simulink library "AEMS_Standard_Library"  (R2016b)
settings: Solver=ode45  StartTime=0.0  StopTime=10.0  RelTol=1e-3
undefined symbols (not defined in the file or in its folder): BkPY, carto, Cbx_extegr, Cbx_lpegrsys, Cbx_portegr, Cnx_bnk_nr_conf, Cnx_cyl_nr_conf, ConfigManagement, configuration_management, Cxx_dcm_io_tmr_end_xxxx, Cxx_dcm_rt_tmr_end, Cxx_DID_xxxx_IO_max, Cxx_DID_xxxx_IO_min, Cxx_egrhsofs, Cxx_vmaniegi, DEM_DEBOUNCE_FREEZE, DEM_DTR_CTL_INVISIBLE, DEM_DTR_CTL_NORMAL, Dem_DtrId2_XXX, Dem_DtrId3_XXX, Dem_DtrId4_XXX, Dem_DtrId5_XXX, Dem_DtrId6_XXX, Dem_DtrId7_XXX, Dem_DtrId8_XXX, Dem_DtrId9_XXX, Dem_DtrId_XXX, Dem_EnableConditionId2_XXX, Dem_EnableConditionId3_XXX, Dem_EnableConditionId4_XXX, Dem_EnableConditionId5_XXX, Dem_EnableConditionId6_XXX, Dem_EnableConditionId7_XXX, Dem_EnableConditionId8_XXX, Dem_EnableConditionId_XXX, Dem_EventId, Dem_EventId2_XXX, Dem_EventId3_XXX, Dem_EventId4_XXX, Dem_EventId5_XXX, Dem_EventId6_XXX, Dem_EventId7_XXX, Dem_EventId8_XXX, Dem_EventId9_XXX, Dem_EventId_Device_Faulttype, Dem_EventId_XXX, DEM_IUMPR_GENERAL_DENOMINATOR, DEM_OPCYC_IGNITION, Dem_RatioId2_XXX, Dem_RatioId3_XXX, Dem_RatioId4_XXX, Dem_RatioId5_XXX, Dem_RatioId6_XXX, Dem_RatioId7_XXX, Dem_RatioId8_XXX, Dem_RatioId_XXX, Dem_StorageConditionId2_XXX, Dem_StorageConditionId3_XXX, Dem_StorageConditionId4_XXX, Dem_StorageConditionId5_XXX ... (+65)
libraries: AEMS_Standard_Library x477, simulink x2
(part 8 of 39)

== system AEMS_Standard_Library/DISCONTINUITIES ==
  AEMS_DEADZONE : Subsystem  Tag=[LIB]  mask(AEMS_DEADZONE){mf=off}
      mask prompts: mf "Curve inflexion dead-zone"
      mask help:
      | Outputs zero for inputs within the dead zone.
      | Offset input signals by either the Start(lowerlimit) or End(upperlimit) value when the input is outside the dead zone.
      |
      | 'Start' is the lower dead-zone boundary.
      | 'End' is the upper dead-zone boundary.
      |
      | For 'Curve inflexion dead-zone' checked OFF, the output signal has three phases based on input signal VALUE:
      |
      | 1] When input signal is below the 'start' boundary, the output signal has an offset of - 'start'.
      | 2] When input signal is above the 'end' boundary, the output signal has an offset of - 'end'.
      | 3] When input signal is between the 'start' and 'end' boundaries, the output signal is set to ZERO
      |
      | For 'Curve inflexion dead-zone' checked ON, the output signal has three phases based on input signal VALUE and its DERIVATIVE (with respect to time):
      |
      | 1] When input signal derivative is positive (and remains positive), the output signal has an offset of - 'start'.
      | 2] When input signal derivative is negative (and remains negative), the output signal has an offset of - 'end'.
      | 3] When input signal derivative changes sign, the output signal keeps its last value until it has an offset of  - 'start' (for a - to + change) or - 'end' (for a + to - change).
      mask init:
      | if mf
      |     patch_out=[0,.1,.4,.6,.8,1,1,.8,.6,.4,.1,0;.19,.19,.49,.49,.29,.29,.31,.31,.51,.51,.21,.21];
      | else
      |     patch_out=[0,.1,.3,.4,.5,.7,.8,.9,1,1,.9,.8,.7,.5,.4,.3,.1,0;.29,.39,.39,.49,.39,.39,.29,.39,.39,.41,.41,.31,.41,.41,.51,.41,.41,.31];
      | end
      settings: AttributesFormatString=%<MaskType>\nCurve inflexion dead-zone = %<mf>
      mask Help:
      | eval('path_lib=fileparts(which(''AEMS_Standard_Library''));');
      | doc_path = [path_lib '\help\AEMS_DEADZONE.pdf'];
      | eval('open(doc_path)');
      mask Display:
      | patch([0,.4,.8,1,1,.8,.4,0],[.19,.59,.19,.39,.41,.21,.61,.21],[0 0 1])
      | 
      | patch(patch_out(1,:),patch_out(2,:),[1 0 0])
      | 
      | 
      | plot([0.02,0.02,0.02])
      | plot([0.98,0.98,0.98])
      | 
      | text(0.5, 0.15, 'AEMS_DEADZONE', 'horizontalAlignment', 'center');
  AEMS_ENUMERATION_SWITCH : Subsystem  Tag=[LIB]  mask(AEMS_ENUMERATION_SWITCH){DataPortIndices={[Nnx_aaa_stt, Nnx_bbb_stt] ,Nnx_ccc_stt,Nnx_ddd_stt}, DataPortForDefault=Last data port}
      mask prompts: DataPortIndices "Data Port Indices"; DataPortForDefault "Data port for default case"
      mask help: Custom multiport switch block to display enum constant names on the mask.
      mask init:
      | % To mask the Multiport Switch block
      | 
      | %% Getting parameter data
      | ThisBlk=gcb;
      | DPI_tmp=get_param(ThisBlk,'DataPortIndices');
      | DPI = regexprep(DPI_tmp,'\s','');
      | DPDC=get_param(ThisBlk,'DataPortForDefault');
      | 
      | %% CHECK PART
      | % If parameters are the same, do nothing
      | Internal_DPI=get_param([ThisBlk '/MultiportSwitch'],'DataPortIndices');
      | Internal_DPDC=get_param([ThisBlk '/MultiportSwitch'],'DataPortForDefault');
      | if strcmp(DPI,Internal_DPI) && strcmp(DPDC,Internal_DPDC) 
      |     return
      | end
      | 
      | % Test if some parameters are in duplicate
      | DPI_complete=strsplit(regexprep(DPI,'{|}|\[|\]',''),',');
      | DPI_unique = unique(DPI_complete,'stable');
      | if ~isequal(DPI_complete,DPI_unique)
      |     msgbox('Invalid setting for data port indices. The same Nnx is used more than once','Error','error');
      |     return
      | end
      | 
      | % Test if some parameters are not Nnx_stt
      | if ~all(startsWith(DPI_complete,'Nnx')) || ~all(endsWith(DPI_complete,'_stt'))
      |     msgbox('Data port indices should start with ''Nnx'' and end with ''stt''','Error','error');
      |     return
      | end
      | 
      | %% MODIFICATION OF INNER PART
      | 
      | 
      | % Total number of inports we need inside incl. default case
      | TargetInports = regexp(DPI,'(\w+)|\[([^\[\]]*)\]','tokens');
      | if isequal(DPDC,'Additional data port')
      |     TargetInports_Nb = numel(TargetInports)+1;
      | else
      |     TargetInports_Nb = numel(TargetInports);
      | end
      | 
      | % Total number of existing inports
      | ExistingInports=find_system(ThisBlk,'LookUnderMasks','all','FollowLinks','on','regexp','on','BlockType','Inport','Name','^Dataport');
      | ExistingInports_Nb = length(ExistingInports);
      | 
      | % If we need to create inports and their lines
      | if TargetInports_Nb > ExistingInports_Nb    
      |         % creating blocks
      |         PreviousInportPosition=get_param([ThisBlk '/Dataport' num2str(ExistingInports_Nb)],'Position');
      |         for num=ExistingInports_Nb:(TargetInports_Nb-1)
      |             NewInportPosition=[10   PreviousInportPosition(2)+35    40   PreviousInportPosition(4)+35];
      |             add_block('built-in/Inport',[ThisBlk '/Dataport' num2str(num+1)],'Position',NewInportPosition,'BackgroundColor','green');
      |             PreviousInportPosition(2)= NewInportPosition(2);
      |             PreviousInportPosition(4)= NewInportPosition(4);
      |         end
      | % If we need to delete inports and their lines
      | elseif TargetInports_Nb < ExistingInports_Nb
      |         for num=(TargetInports_Nb):ExistingInports_Nb-1
      |             delete_block([ThisBlk '/Dataport' num2str(num+1)]);
      |         end
      | end
      | 
      | % We set the parameters of the inner block to the new ones
      | % Script may fail here if a data is not defined
      | try
      |     set_param([ThisBlk,'/MultiportSwitch'],'DataPortForDefault',DPDC,'DataPortIndices',DPI);
      | 
      |     % deleting all lines then creating all lines
      |     delete_line(find_system(ThisBlk,'FindAll','on','FollowLinks','on','LookUnderMasks','all','Type','line'));
      |     add_line(ThisBlk,'Control_Input/1','MultiportSwitch/1','Autorouting','On');
      |     add_line(ThisBlk,'MultiportSwitch/1','Out/1','Autorouting','On');
      |     for num=0:(TargetInports_Nb-1)
      |         add_line(ThisBlk,['Dataport' num2str(num+1) '/1'],['MultiportSwitch/' num2str(num+2)],'Autorouting','On');
      |     end
      | catch
      | end
      settings: AttributesFormatString=%<MaskType>\nData port for default case = %<DataPortForDefault>
      mask Help:
      | eval('path_lib=fileparts(which(''AEMS_Standard_Library''));');
      | doc_path = [path_lib '\help\AEMS_ENUMERATION_SWITCH.pdf'];
      | eval('open(doc_path)');
      mask TypeOptions DataPortForDefault: Last data port | Additional data port
      mask Display:
      | % To mask the Multiport Switch block
      | 
      | %% Getting parameter data
      | ThisBlk=gcb;
      | DPI = get_param(ThisBlk,'DataPortIndices');
      | DPI = regexprep(DPI,'\s','');
      | DPDC=get_param(ThisBlk,'DataPortForDefault');
      | 
      | 
      | %% CHECK PART
      | % Test if some parameters are in duplicate
      | DPI_complete=strsplit(regexprep(DPI,'{|}|\[|\]',''),',');
      | DPI_unique = unique(DPI_complete,'stable');
      | if ~isequal(DPI_complete,DPI_unique)
      |    disp('!!! Invalid Settings !!!\nDuplicate Nnx');
      |    return
      | end
      | 
      | % Test if some parameters are not Nnx_stt
      | if ~all(startsWith(DPI_complete,'Nnx')) || ~all(endsWith(DPI_complete,'_stt'))
      |    disp('!!! Invalid Settings !!!\nNot all Nnx_..._stt constants');
      |    return
      | end
      | 
      | 
      | %%DRAWING PART
      | Blkpos = get_param(ThisBlk,'Position');
      | PortHandles=get_param(gcb,'PortHandles');
      | IPort_Pos=get_param(PortHandles.Inport,'Position');
      | BlockHeightPx = Blkpos(4)-Blkpos(2);
      | 
      | %% drawing inputs
      | % splitting fileds in inputs
      | Inputs_ToDraw = regexp(DPI,'(\w+)|\[([^\[\]]*)\]','tokens');
      | 
      | % adding carriage returns every two Nnx in case there in several per input,
      | % and spaces after each comma
      | Inputs_ToDraw=cellfun(@(x) regexprep(x,'(\w+\,\w+\,)','$1\n'),Inputs_ToDraw,'UniformOutput',0);
      | Inputs_ToDraw=cellfun(@(x) regexprep(x,'(\w+)\,','$1, '),Inputs_ToDraw,'UniformOutput',0);
      | 
      | Input_YPos=cellfun(@(x) (Blkpos(4)-x(2))/BlockHeightPx,IPort_Pos,'UniformOutput',0);
      | for i=2:(numel(Input_YPos))
      |     x=[-0.1,0.4];
      |     y=[Input_YPos{i},Input_YPos{i}];
      |     plot(x,y);
      | 
      |     if i==numel(Input_YPos)
      |         if isequal(DPDC,'Additional data port')
      |             port_label('input', i, ['*' sprintf('\n')]);
      |         else
      |             port_label('input', i, ['*, ' char(Inputs_ToDraw{i-1}) sprintf('\n')]);
      |         end
      |     else
      |         port_label('input', i, [char(Inputs_ToDraw{i-1}) sprintf('\n')]);
      |     end
      | end
      | 
      | %% draw selector lines
      | x=[-0.1 0.3];
      | y=[Input_YPos{1},Input_YPos{1}];
      | plot(x,y);
      | x=[0.3,0.3];
      | y=[Input_YPos{1}+0.04,Input_YPos{1}-0.04];
      | plot(x,y);
      | 
      | %% draw output lines
      | XPlot_Line = [0.43,0.8,1.1];
      | YPlot_Line = [Input_YPos{2},0.5,0.5];
      | plot(XPlot_Line,YPlot_Line);
  AEMS_MULTI_PORT_TIME_SWITCH : Subsystem  Tag=[LIB]  mask(AEMS_MULTI_PORT_TIME_SWITCH){}
      mask help:
      | This switch allows the user to switch among 8 input signals using the Vsx_sel input. It provides a smooth transition between the previously selected signal and the currently selected signal over a period of time, set by Vxx_swi_t.
      |
      | It should be noted that during the transition, the current value of both signals is taken into account and not just values at the moment of switching.
      |
      | As a result, discontinuities can arise if a new signal is seleted before the previous transition has ended.
      settings: AttributesFormatString=%<MaskType>
      mask Help:
      | eval('path_lib=fileparts(which(''AEMS_Standard_Library''));');
      | doc_path = [path_lib '\help\AEMS_MULTI_PORT_TIME_SWITCH.pdf'];
      | eval('open(doc_path)')
      mask Display: disp('AEMS_MULTI_PORT_TIME_SWITCH')
  AEMS_SLEW_RATE : Subsystem  Tag=[LIB]  mask(AEMS_SLEW_RATE){}
      mask help:
      | This block is a Slew rate block, which limits the increase and decrease of the INPUT by using calibrated slopes independent of sampling time.
      | POS_SLOPE : positive maximum slope parameter per second.
      | NEG_SLOPE : negative maximum slope parameter per second.
      |
      | Reference to AUTOSAR specification:
      | AUTOSAR Service Name : Mfl_RampCalc
      | Reference : SWS_Mfl_00201
      settings: AttributesFormatString=%<MaskType>
      mask Help:
      | eval('path_lib=fileparts(which(''AEMS_Standard_Library''));');
      | doc_path = [path_lib '\help\AEMS_SLEW_RATE.pdf'];
      | eval('open(doc_path)')
      mask Display:
      | patch([0.1 0.2 0.22 0.25 0.3 0.35 0.4 0.45 0.5 0.6 0.6 0.5 0.45 0.4 0.35 0.3 0.25 0.22 0.2 0.1],[0.24 0.24 0.34 0.44 0.59 0.69 0.79 0.84 0.89 0.89 0.93 0.93 0.88 0.83 0.73 0.63 0.48 0.38 0.28 0.28],[0 0 1]);
      | patch([0.5 0.6 0.65 0.68 0.72 0.79 0.8 0.9 0.9 0.8 0.79 0.72 0.68 0.65 0.6 0.5],[0.89 0.89 0.76 0.71 0.67 0.65 0.64 0.64 0.68 0.68 0.69 0.71 0.75 0.8 0.93 0.93],[0 0 1])
      | patch([0.1 0.2 0.5 0.6 0.8 0.9 0.9 0.8 0.6 0.5 0.2 0.1],[0.25 0.25 0.9 0.9 0.65 0.65 0.67 0.67 0.92 0.92 0.27 0.27],[1 0 0]);
  AEMS_SLOPE_SWITCH : Subsystem  Tag=[LIB]  mask(AEMS_SLOPE_SWITCH){}
      mask help:
      | This block is a Multiple Port Slope Switch.
      | Depending on the value of input Switch_Cmd (from 0), the block outputs the corresponding input signal.
      | For Switch_Cmd = 0, Output is In0, for Switch_Cmd = 1, Output is In1, and so on...
      |
      | Nevertheless, for each switch between two input signals, a slope is activated from the first input signal to the second input signal.
      | The value of this slope is given by Pos_Slope if the input signal to reach is over the initial input signal and by Neg_Slope if the input signal to reach is under.
      | Pos_Slope and Neg_Slope are respectively the positive and negative slope parameters per second.
      |
      | The output Slope_On indicates if a transition is active (Slope_On at true) or not (Slope_On at false).
      settings: AttributesFormatString=%<MaskType>
      mask Help:
      | eval('path_lib=fileparts(which(''AEMS_Standard_Library''));');
      | doc_path = [path_lib '\help\AEMS_SLOPE_SWITCH.pdf'];
      | eval('open(doc_path)')
      mask Display:
      | color ('blue')
      | disp('SLOPE SWITCH\n\n 2 INPUTS')
  AEMS_SLOPE_SWITCH_3INPUTS : Subsystem  Tag=[LIB]  mask(AEMS_SLOPE_SWITCH_3INPUTS){}
      mask help:
      | This block is a Multiple Port Slope Switch.
      | Depending on the value of input Switch_Cmd (from 0), the block outputs the corresponding input signal.
      | For Switch_Cmd = 0, Output is In0, for Switch_Cmd = 1, Output is In1, and so on...
      |
      | Nevertheless, for each switch between two input signals, a slope is activated from the first input signal to the second input signal.
      | The value of this slope is given by Pos_Slope if the input signal to reach is over the initial input signal and by Neg_Slope if the input signal to reach is under.
      | Pos_Slope and Neg_Slope are respectively the positive and negative slope parameters per second.
      |
      | The output Slope_On indicates if a transition is active (Slope_On at true) or not (Slope_On at false).
      settings: AttributesFormatString=%<MaskType>
      mask Help:
      | eval('path_lib=fileparts(which(''AEMS_Standard_Library''));');
      | mskblk=get_param(gcbh,'MaskType');
      | doc_path = [path_lib '\help\',mskblk,'.pdf'];
      | eval('open(doc_path)');
      mask Display:
      | color ('blue')
      | disp('SLOPE SWITCH\n\n 3 INPUTS')
  AEMS_SLOPE_SWITCH_4INPUTS : Subsystem  Tag=[LIB]  mask(AEMS_SLOPE_SWITCH_4INPUTS){}
      mask help:
      | This block is a Multiple Port Slope Switch.
      | Depending on the value of input Switch_Cmd (from 0), the block outputs the corresponding input signal.
      | For Switch_Cmd = 0, Output is In0, for Switch_Cmd = 1, Output is In1, and so on...
      |
      | Nevertheless, for each switch between two input signals, a slope is activated from the first input signal to the second input signal.
      | The value of this slope is given by Pos_Slope if the input signal to reach is over the initial input signal and by Neg_Slope if the input signal to reach is under.
      | Pos_Slope and Neg_Slope are respectively the positive and negative slope parameters per second.
      |
      | The output Slope_On indicates if a transition is active (Slope_On at true) or not (Slope_On at false).
      settings: AttributesFormatString=%<MaskType>
      mask Help:
      | eval('path_lib=fileparts(which(''AEMS_Standard_Library''));');
      | doc_path = [path_lib '\help\AEMS_SLOPE_SWITCH_4INPUTS.pdf'];
      | eval('open(doc_path)')
      mask Display:
      | color ('blue')
      | disp('SLOPE SWITCH\n\n 4 INPUTS')
  AEMS_SLOPE_SWITCH_6INPUTS : Subsystem  Tag=[LIB]  mask(AEMS_SLOPE_SWITCH_6INPUTS){}
      mask help:
      | This block is a Multiple Port Slope Switch.
      | Depending on the value of input Switch_Cmd (from 0), the block outputs the corresponding input signal.
      | For Switch_Cmd = 0, Output is In0, for Switch_Cmd = 1, Output is In1, and so on...
      |
      | Nevertheless, for each switch between two input signals, a slope is activated from the first input signal to the second input signal.
      | The value of this slope is given by Pos_Slope if the input signal to reach is over the initial input signal and by Neg_Slope if the input signal to reach is under.
      | Pos_Slope and Neg_Slope are respectively the positive and negative slope parameters per second.
      |
      |
      | The output Slope_On indicates if a transition is active (Slope_On at true) or not (Slope_On at false).
      settings: AttributesFormatString=%<MaskType>
      mask Help:
      | eval('path_lib=fileparts(which(''AEMS_Standard_Library''));');
      | mskblk=get_param(gcbh,'MaskType');
      | doc_path = [path_lib '\help\',mskblk,'.pdf'];
      | eval('open(doc_path)');
      mask Display:
      | color ('blue')
      | disp('SLOPE SWITCH\n\n 6 INPUTS')
  AEMS_SLOPE_SWITCH_8INPUTS : Subsystem  Tag=[LIB]  mask(AEMS_SLOPE_SWITCH_8INPUTS){}
      mask help:
      | This block is a Multiple Port Slope Switch.
      | Depending on the value of input Switch_Cmd (from 0), the block outputs the corresponding input signal.
      | For Switch_Cmd = 0, Output is In0, for Switch_Cmd = 1, Output is In1, and so on...
      |
      | Nevertheless, for each switch between two input signals, a slope is activated from the first input signal to the second input signal.
      | The value of this slope is given by Pos_Slope if the input signal to reach is over the initial input signal and by Neg_Slope if the input signal to reach is under.
      | Pos_Slope and Neg_Slope are respectively the positive and negative slope parameters per second.
      |
      |
      | The output Slope_On indicates if a transition is active (Slope_On at true) or not (Slope_On at false).
      settings: AttributesFormatString=%<MaskType>
      mask Help:
      | eval('path_lib=fileparts(which(''AEMS_Standard_Library''));');
      | doc_path = [path_lib '\help\AEMS_SLOPE_SWITCH_8INPUTS.pdf'];
      | eval('open(doc_path)')
      mask Display:
      | color ('blue')
      | disp('SLOPE SWITCH\n\n 8 INPUTS')

== system AEMS_Standard_Library/DISCRETE ==
  AEMS_UNITDELAY_EXTERNALIC : Subsystem  Tag=[LIB]  mask(AEMS_UNITDELAY_EXTERNALIC){}
      mask help:
      | The input signal (u) signal will be delayed by one sample period and given as output (y).
      | Initial condition is given by the signal IC.
      |
      | Note: Input must be without offset
      settings: AttributesFormatString=%<MaskType>
      mask Help:
      | eval('path_lib=fileparts(which(''AEMS_Standard_Library''));');
      | doc_path = [path_lib '\help\AEMS_UNITDELAY_EXTERNALIC.pdf'];
      | eval('open(doc_path)')
      mask Display: dpoly(1,[1 0],'z')
  AEMS_UNITDELAY_RESET_EXTERNALIC : Subsystem  Tag=[LIB]  mask(AEMS_UNITDELAY_RESET_EXTERNALIC){}
      mask help:
      | The output is the signal (u) delayed by one sample period.
      | When the reset signal 'R' is true, the state and the output are always set equal to the initial condition signal 'IC'.  This reset action is vectorized and supports scalar expansion.
      settings: AttributesFormatString=%<MaskType>
      mask Help:
      | eval('path_lib=fileparts(which(''AEMS_Standard_Library''));');
      | doc_path = [path_lib '\help\AEMS_UNITDELAY_RESET_EXTERNALIC.pdf'];
      | eval('open(doc_path)')
      mask Display: dpoly(1,[1 0],'z')

== system AEMS_Standard_Library/EDGE ==
  AEMS_EDGE_EITHER : Subsystem  Tag=[LIB]  mask(AEMS_EDGE_EITHER){init=false}
      mask prompts: init "Initial Value of Input"
      mask help:
      | This block can be used to :
      |
      | Detect change   - If the input signal(In) is changing from '0' to '1' OR '1' to '0'
      |
      | The initial value of Input is given in the mask. By default it gets value FALSE.
      |
      | The output is a signal of data type 'boolean'.
      |
      | Reference to AUTOSAR specification:
      |         AUTOSAR Service Name :  Efx_EdgeBipol_u8_u8
      |         Reference : SWS_Efx_00380
      mask init:
      | a=0.2;
      | b=0.4;
      | c=0.6;
      | d=0.9;
      | e=0.6;
      | f=0.6;
      | g=0.9;
      | if strcmp(init,'false')
      |    InitValue=0;
      | elseif strcmp(init,'true')
      |    InitValue=1; 
      | end
      settings: AttributesFormatString=|
      | %<MaskType>
      | Initial Value : %<init>
      mask Help:
      | eval('path_lib=fileparts(which(''AEMS_Standard_Library''));');
      | mskblk=get_param(gcbh,'MaskType');
      | doc_path = [path_lib '\help\',mskblk,'.pdf'];
      | eval('open(doc_path)');
      mask TypeOptions init: false | true
      mask DialogControl DescGroupVar_copy Prompt: Initialization
      mask Display:
      | color('green');
      | plot([a b b c],[f f g g]);
      | color('red');
      | plot([a b b c],[d d e e]);
      | color('blue');
      | plot([a b b b c],[0.1 0.1 0.4 0.1 0.1])
  AEMS_EDGE_FALLING : Subsystem  Tag=[LIB]  mask(AEMS_EDGE_FALLING){init=false}
      mask prompts: init "Initial Value of Input"
      mask help:
      | This block can be used to :
      |
      | Detect decrease - If the input signal(In) is changing from '1' to '0'.
      |
      | The initial value of Input is given in the mask. By default it gets value FALSE.
      |
      | The output is a signal of data type 'boolean'.
      |
      | Reference to AUTOSAR specification:
      |          AUTOSAR Service Name :  Efx_EdgeFalling_u8_u8
      |          Reference : SWS_Efx_00382
      mask init:
      | a=0.2;
      | b=0.4;
      | c=0.6;
      | d=0.9;
      | e=0.6;
      | f=0.9;
      | g=0.6;
      | if strcmp(init,'false')
      |    InitValue=0;
      | elseif strcmp(init,'true')
      |    InitValue=1; 
      | end
      settings: AttributesFormatString=|
      | %<MaskType>
      | Initial Value : %<init>
      mask Help:
      | eval('path_lib=fileparts(which(''AEMS_Standard_Library''));');
      | mskblk=get_param(gcbh,'MaskType');
      | doc_path = [path_lib '\help\',mskblk,'.pdf'];
      | eval('open(doc_path)');
      mask TypeOptions init: false | true
      mask Display:
      | color('green');
      | plot([a b b c],[f f g g]);
      | color('red');
      | plot([a b b c],[d d e e]);
      | color('blue');
      | plot([a b b b c],[0.1 0.1 0.4 0.1 0.1])
  AEMS_EDGE_RISING : Subsystem  Tag=[LIB]  mask(AEMS_EDGE_RISING){init=false}
      mask prompts: init "Initial Value of Input"
      mask help:
      | This block can be used to :
      |
      | Detect increase - If the input signal(In) is changing from '0' to '1'.
      |
      | The initial value of Input is given in the mask. By default it gets value FALSE.
      |
      | The output is a signal of data type 'boolean'.
      |
      | Reference to AUTOSAR specification:
      |         AUTOSAR Service Name :  Efx_EdgeRising_u8_u8
      |         Reference : SWS_Efx_00384
      mask init:
      | %Rising
      | a=0.2;
      | b=0.4;
      | c=0.6;
      | d=0.6;
      | e=0.9;
      | f=0.6;
      | g=0.9;
      | if strcmp(init,'false')
      |    InitValue=0;
      | elseif strcmp(init,'true')
      |    InitValue=1; 
      | end
      settings: AttributesFormatString=|
      | %<MaskType>
      | Initial Value : %<init>
      mask Help:
      | eval('path_lib=fileparts(which(''AEMS_Standard_Library''));');
      | mskblk=get_param(gcbh,'MaskType');
      | doc_path = [path_lib '\help\',mskblk,'.pdf'];
      | eval('open(doc_path)');
      mask TypeOptions init: false | true
      mask Display:
      | color('green');
      | plot([a b b c],[f f g g]);
      | color('red');
      | plot([a b b c],[d d e e]);
      | color('blue');
      | plot([a b b b c],[0.1 0.1 0.4 0.1 0.1])

== system AEMS_Standard_Library/FILTER ==
  AEMS_DISCRETE_TIME_INTEGRATOR_EULER : Subsystem  Tag=[LIB]  mask(AEMS_DISCRETE_TIME_INTEGRATOR_EULER){Upper_limit=255, Lower_limit=0}
      mask prompts: Upper_limit "Upper Saturation Limt"; Lower_limit "Lower Saturation Limit"
      mask help:
      | The block can integrate or accumulate using the Forward Euler.
      | The resulting expression for the output of the block at step n is
      | y(n) = x(n-1)*T*K + y(n-1)
      settings: AttributesFormatString=%<MaskType>\nUpper Saturation Limit = %<Upper_limit>\nLower Saturation Limit = %<Lower_limit>
      mask Help:
      | eval('path_lib=fileparts(which(''AEMS_Standard_Library''));');
      | doc_path = [path_lib '\help\AEMS_DISCRETE_TIME_INTEGRATOR_EULER.pdf'];
      | eval('open(doc_path)')
      mask Display: disp('Discrete-Time \n Integrator')
  AEMS_FILTER_WITH_DELAY_CONTROL : Subsystem  Tag=[LIB]  mask(AEMS_FILTER_WITH_DELAY_CONTROL){}
      mask help:
      | The principle of this filter is based on slopes limitation of the signal to process.
      | The set points to limit the negative and positive slopes are computed with the derivate of the input filtered signal using a low pass first order filter.
      | The set points are then fixed by a proportional integrator controller in order to minimize the error between the input and output.
      |
      | Notes: filter_param is calculated from time constant and sample time as:
      | filter_param=1-exp(-T/Tau) where T is sample time and Tau is time constant.
      |
      | See Help document for more information.
      settings: AttributesFormatString=%<MaskType>
      mask Help:
      | eval('path_lib=fileparts(which(''AEMS_Standard_Library''));');
      | doc_path = [path_lib '\help\AEMS_FILTER_WITH_DELAY_CONTROL.pdf'];
      | eval('open(doc_path)')
      mask Display:
      | port_label('input',1,'filter_param')
      | port_label('input',2,'kp')
      | port_label('input',3,'Input')
      | port_label('input',4,'timestep')
      | port_label('output',1,'Output')
      | disp('AEMS_FILTER_WITH_DELAY_CONTROL')
  AEMS_FIRST_ORDER_FILTER_RST : Subsystem  Tag=[LIB]  mask(AEMS_FIRST_ORDER_FILTER_RST){}
      mask help:
      | This block is a First-Order Filter, with :
      | 	- Filter_param: filter parameter calculated from time constant and sample time.
      | 	- IC the initial value.
      | 	- R the reset signal.
      | The initial condition is given by the signal IC.
      | When the reset signal is true, output is set equal to the initial condition signal IC.
      |
      | Notes: Filter_param is calculated from time constant and sample time as:
      | Filter_param=1-exp(-T/Tau) where T is sample time and Tau is time constant.
      |
      | Reference to AUTOSAR specification:
      | -	AUTOSAR Service Name:  Efx_LpFilter
      | -	Reference: [SWS_Efx_00012]
      |
      | See Help document for more information.
      settings: AttributesFormatString=%<MaskType>
      mask Help:
      | eval('path_lib=fileparts(which(''AEMS_Standard_Library''));');
      | mskblk=get_param(gcbh,'MaskType');
      | doc_path = [path_lib '\help\',mskblk,'.pdf'];
      | eval('open(doc_path)');
      mask Display:
      | plot([0.2  0.2],[0.1 0.9 ]);
      | plot([0.25  0.2],[0.8 0.9 ]);
      | plot([0.15  0.2],[0.8 0.9 ]);
      | plot([0.9  0.2],[0.8 0.8 ]);
      | plot([0.2  1],[0.1 0.1 ]);
      | plot([0.2:0.01:0.85],0.1+0.7-0.7*exp(5*[0:-0.01:-.65]));
      | plot([1  0.9],[0.1 0.15]);
      | plot([1  0.9],[0.1 0.05]);
  AEMS_FORWARD_EULER_INTEGRATOR_WITH_RESET : Subsystem  Tag=[LIB]  mask(AEMS_FORWARD_EULER_INTEGRATOR_WITH_RESET){}
      mask help:
      | This block will perform discrete-time integration or accumulation of input signal based on Euler's method :
      | y[k] = y[k-1] + K.Ts.u[k-1]
      |
      |  Where,
      |  K = gain
      |  Ts = sample time.
      |  IC = initial condition.
      |
      | Output(y) will be limited by upper and lower saturation limits. Resets the state when the reset signal rises or falls.
      settings: AttributesFormatString=%<MaskType>
      mask Help:
      | eval('path_lib=fileparts(which(''AEMS_Standard_Library''));');
      | doc_path = [path_lib '\help\AEMS_FORWARD_EULER_INTEGRATOR_WITH_RESET.pdf'];
      | eval('open(doc_path)')
  AEMS_TAU_TO_FILTER_PARAM : Subsystem  Tag=[LIB]  mask(AEMS_TAU_TO_FILTER_PARAM){Nxb_fil_para=Nxb_fil_para, Nxp_fil_para=Nxp_fil_para}
      mask prompts: Nxb_fil_para "Breakpoint"; Nxp_fil_para "Map"
      mask help:
      | This bloc is to calculate filter parameter by interpolation from time constant and time step.
      |
      | -INPUTS-
      | Timestep: Time step
      | Tau: Time constant of filter
      |
      | -OUTPUTS-
      | Filter_param: Filter parameter Filter_param=exp(-Timestep/Tau).
      |
      | -PARAMETERS-
      | Breakpoint: break points of exponential function, defined in Nxb_fil_para by default
      | Map: map of exponential function, defined in Nxp_fil_para by default
      settings: AttributesFormatString=|
      | %<MaskType>
      | Breakpoint: %<Nxb_fil_para>
      | Map: %<Nxp_fil_para>
      mask Help:
      | eval('path_lib=fileparts(which(''AEMS_Standard_Library''));');
      | doc_path = [path_lib '\help\AEMS_TAU_TO_FILTER_PARAM.pdf'];
      | eval('open(doc_path)')
  AEMS_TAU_TO_FILTER_PARAM_EXP : Subsystem  Tag=[LIB]  mask(AEMS_TAU_TO_FILTER_PARAM_EXP){}
      mask help:
      | This bloc is to calculate filter parameter by interpolation from time constant and time step.
      |
      | -INPUTS-
      | Timestep: Time step
      | Tau: Time constant of filter
      |
      | -OUTPUTS-
      | Filter_param: Filter parameter Filter_param=exp(-Timestep/Tau).
      |
      | -PARAMETERS-
      | Breakpoint: break points of exponential function, defined in Nxb_fil_para by default
      | Map: map of exponential function, defined in Nxp_fil_para by default
      settings: AttributesFormatString=%<MaskType>
      mask Help:
      | eval('path_lib=fileparts(which(''AEMS_Standard_Library''));');
      | doc_path = [path_lib '\help\AEMS_TAU_TO_FILTER_PARAM_EXP.pdf'];
      | eval('open(doc_path)')
      mask Display: disp('Obsolete\n Do not use for\nnew design')

== system AEMS_Standard_Library/FLAG ==
  AEMS_SRFLIPFLOP : Subsystem  Tag=[LIB]  mask(AEMS_SRFLIPFLOP){init=false}
      mask prompts: init "Initial condition (state of Q):"
      mask help:
      | S-R Flip-Flop Block
      | The S-R flip-flop also known as a reset-set flip-flop. This block is
      | designed using NOR gates. The truth table for this block is found below:
      |
      |  S  R  Q
      |  -----------
      |  0  0   Q
      |  0  1   0
      |  1  0   1
      |  1  1   0
      |
      | In an S-R flip-flop that is implemented with NOR gates, when a 1 is
      | applied to both the set and reset inputs, output goes to 0. Technically,
      | this state is undefined and is usually avoided.
      |
      | Reference to AUTOSAR specification:
      |         AUTOSAR Service Name :  Efx_RSFlipFlop
      |         Reference : SWS_Efx_00405
      mask init:
      | if strcmp(init,'false')
      |    InitValue=0;
      | elseif strcmp(init,'true')
      |    InitValue=1; 
      | end
      settings: AttributesFormatString=%<MaskType>\nInitial condition (state of Q): = %<init>
      mask Help:
      | eval('path_lib=fileparts(which(''AEMS_Standard_Library''));');
      | mskblk=get_param(gcbh,'MaskType');
      | doc_path = [path_lib '\help\',mskblk,'.pdf'];
      | eval('open(doc_path)');
      mask TypeOptions init: false | true

== system AEMS_Standard_Library/HYSTERESIS ==
  AEMS_HYST_DELTARIGHT : Subsystem  Tag=[LIB]  mask(AEMS_HYST_DELTARIGHT){}
      mask help:
      | Hysteresis Function
      |
      | Hys Type  :  Minus
      | Lower Threshold  :  Not Included
      | Upper Threshold  :  Not Included
      | Lower Hys Flag Value  :  0
      | Upper Hys Flag Value  :  1
      |
      | I/O
      | val     :  Value
      | thrs    :  Right Threshold Value
      | hysw  :  Hysteresis Width
      |
      | flg_ret  :  Answer Flag Value
      |
      | set   : val > thrs
      | clear : val < thrs - hysw
      |
      | Reference to AUTOSAR specification:
      |         AUTOSAR Service Name :  Mfl_HystDeltaRight_f32_u8
      |         Reference : SWS_Mfl_00246
      settings: AttributesFormatString=%<MaskType>
      mask Help:
      | eval('path_lib=fileparts(which(''AEMS_Standard_Library''));');
      | mskblk=get_param(gcbh,'MaskType');
      | doc_path = [path_lib '\help\',mskblk,'.pdf'];
      | eval('open(doc_path)');
  AEMS_HYST_LEFTDELTA : Subsystem  Tag=[LIB]  mask(AEMS_HYST_LEFTDELTA){}
      mask help:
      | Left Delta Hysteresis Function
      |
      | Lower Threshold  :  Not Included
      | Upper Threshold  :  Not Included
      | Lower Hys Flag Value  :  0
      | Upper Hys Flag Value  :  1
      |
      | I/O
      | val     :  Value
      | thrs    :  Left Threshold Value
      | hysw  :  Hysteresis Width
      |
      | flg_ret  :  Answer Flag Value
      |
      | set   : val > thrs + hysw
      | clear : val < thrs
      |
      | Reference to AUTOSAR specification:
      |         AUTOSAR Service Name :  Mfl_HystLeftDelta_f32_u8
      |         Reference : SWS_Mfl_00251
      settings: AttributesFormatString=%<MaskType>
      mask Help:
      | eval('path_lib=fileparts(which(''AEMS_Standard_Library''));');
      | mskblk=get_param(gcbh,'MaskType');
      | doc_path = [path_lib '\help\',mskblk,'.pdf'];
      | eval('open(doc_path)');
  AEMS_HYST_LEFTRIGHT : Subsystem  Tag=[LIB]  mask(AEMS_HYST_LEFTRIGHT){init=false, Th1_Strict=off, Th2_Strict=off}
      mask prompts: init "Initial Value of Output"; Th1_Strict "Output false when Input falls to Low_Threshold"; Th2_Strict "Output true when Input increases to High_Threshold"
      mask help:
      | Hysteresis with left and right switching point
      |
      | This block outputs 'false' if 'Input' is < 'Low_Threshold', and 'true' if 'Input' is > 'High_Threshold'. Between these two values, The output will not change, It retains the previoius output value.
      |
      | At the first sample time, if the input is in between the 'Low_Threshold' and 'High_Threshold', output will be the Initial Value.
      |
      | Reference to AUTOSAR specification:
      |         AUTOSAR Service Name : Mfl_HystLeftRight_f32_u8
      |         Reference : SWS_Mfl_00241
      mask init:
      | InitValue=0;
      | if strcmp(init,'false')
      |    InitValue=0;
      | elseif strcmp(init,'true')
      |    InitValue=1; 
      | end
      | dot_x = [-0.02 -0.014 0 0.014 0.02 0.014 0 -0.014 -0.02];
      | dot_y = [0 0.014 0.02 0.014 0 -0.014 -0.02 -0.014 0];
      | Val1 = 0.2; 
      | Val2 = 0.82;
      | Open_T1 = dot_y + Val2;
      | Closed_T1 = dot_y + Val1;
      | Open_T2 = dot_y + Val1;
      | Closed_T2 = dot_y + Val2-0.01;
      | Path_y = [Val1 Val1 Val2 Val2];
      | Real_Opt = find_system(gcb,'SearchDepth',2,'FollowLinks','on','LookUnderMasks','all','BlockType','RelationalOperator');
      | if(Th1_Strict)
      |     Th1_falling='V1';
      |     Th1_V1 = 1;
      |     Th1_V2 = 0;
      |     Open_T1 = dot_y + Val2;
      |     Closed_T1 = dot_y + Val1;
      |     Fall_path_x = [0.2 0.4 0.43 0.8];
      |     Fall_arrow_x = [0.39 0.41 0.43];
      |     set_param(Real_Opt{1},'Operator','>=');
      | else
      |     Th1_falling='V2';
      |     Th1_V1 = 0;
      |     Th1_V2 = 1;
      |     Open_T1 = dot_y + Val1;
      |     Closed_T1 = dot_y + Val2-0.01;
      |     Fall_path_x = [0.2 0.37 0.4 0.8];
      |     Fall_arrow_x = [0.36 0.38 0.40];
      |     set_param(Real_Opt{1},'Operator','>');
      | end
      | if(Th2_Strict)
      |     Th2_rising='V2';
      |     Th2_V1 = 0;
      |     Th2_V2 = 1;
      |     Open_T2 = dot_y + Val1;
      |     Closed_T2 = dot_y + Val2-0.01;
      |     Rise_path_x = [0.2 0.57 0.6 0.8];
      |     Rise_arrow_x = [0.57 0.59 0.61];
      |     set_param(Real_Opt{2},'Operator','>=');
      | else
      |     Th2_rising='V1';
      |     Th2_V1 = 1;
      |     Th2_V2 = 0;
      |     Open_T2 = dot_y + Val2;
      |     Closed_T2 = dot_y + Val1;
      |     Rise_path_x = [0.23 0.6 0.63 0.8];
      |     Rise_arrow_x = [0.6 0.62 0.64];
      |      set_param(Real_Opt{2},'Operator','>');
      | end
      settings: AttributesFormatString=%<MaskType>\nOutput false when Input falls to Threshold 1: %<Th1_Strict>\nOutput true when Input increases to Threshold 2: %<Th2_Strict>\nInitial Value = %<init>
      mask Help:
      | eval('path_lib=fileparts(which(''AEMS_Standard_Library''));');
      | mskblk=get_param(gcbh,'MaskType');
      | doc_path = [path_lib '\help\',mskblk,'.pdf'];
      | eval('open(doc_path)');
      mask TypeOptions init: false | true
      mask Display:
      | % disp(['AEMS_HYSTERESIS' char(10) char(10) char(10) char(10) char(10) char(10) char(10) char(10) char(10)])
      | 
      | plot(Fall_path_x,Path_y,Rise_path_x,Path_y)
      | 
      | plot(Fall_arrow_x,[0.45 0.4 0.45])
      | plot(Rise_arrow_x,[0.55 0.6 0.55])
      | 
      | plot(dot_x+0.4,Open_T1)
      | patch(dot_x+0.4,Closed_T1,[0 0 0])
      | 
      | plot(dot_x+0.6,Open_T2)
      | patch(dot_x+0.6,Closed_T2,[0 0 0])
      | 
      | disp([char(10) char(10)   '         T1      T2' char(10) char(10)])
      | disp([ char(10) char(10) char(10) char(10) char(10) ' false                           '])
      | disp(['                           true'  char(10) char(10) char(10) char(10) char(10) char(10) char(10)])
